simulink model "W06_P1"  (R2024b)
settings: Solver=ode4  StartTime=0  StopTime=T_final  FixedStep=h  RelTol=1e-3
undefined symbols (not defined in the file or in its folder): beta_c, mp, N_SEQ, rp, T_SW, V_c, x0, X_SEQ
settings Model: Creator=admin  LastModifiedBy=admin
settings DataIOCC: ReturnWorkspaceOutputs=off

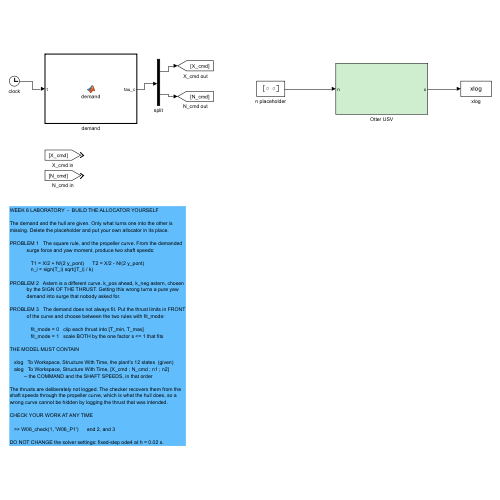
[thumbnail: Simulink's stored preview of the top-level diagram]
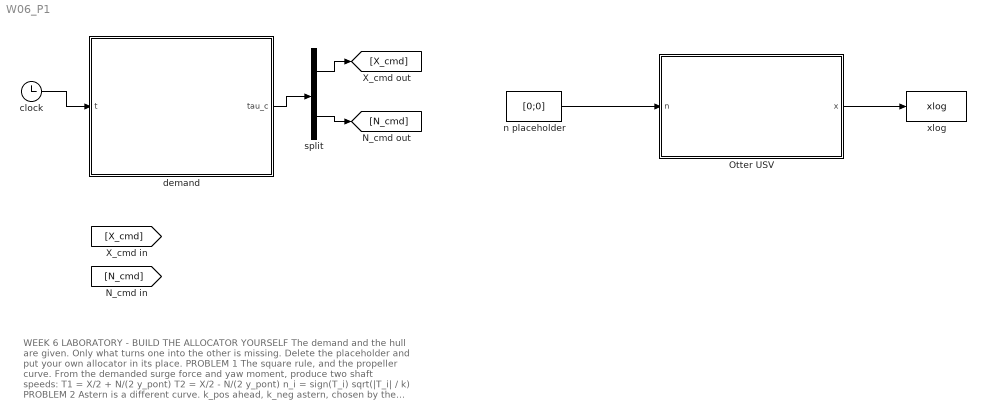
== system W06_P1 ==
  note: WEEK 6 LABORATORY  -  BUILD THE ALLOCATOR YOURSELF
      |
      | The demand and the hull are given. Only what turns one into the other is
      | missing. Delete the placeholder and put your own allocator in its place.
      |
      | PROBLEM 1   The square rule, and the propeller curve. From the demanded
      |             surge force and yaw moment, produce two shaft speeds:
      |
      |                T1 = X/2 + N/(2 y_pont)      T2 = X/2 - N/(2 y_pont)
      |                n_i = sign(T_i) sqrt(|T_i| / k)
      |
      | PROBLEM 2   Astern is a different curve. k_pos ahead, k_neg astern, chosen
      |             by the SIGN OF THE THRUST. Getting this wrong turns a pure yaw
      |             demand into surge that nobody asked for.
      |
      | PROBLEM 3   The demand does not always fit. Put the thrust limits in FRONT
      |             of the curve and choose between the two rules with fit_mode:
      |
      |                fit_mode = 0   clip each thrust into [T_min, T_max]
      |                fit_mode = 1   scale BOTH by the one factor s <= 1 that fits
      |
      | THE MODEL MUST CONTAIN
      |
      |    xlog   To Workspace, Structure With Time, the plant's 12 states  (given)
      |    alog   To Workspace, Structure With Time, [X_cmd ; N_cmd ; n1 ; n2]
      |           -- the COMMAND and the SHAFT SPEEDS, in that order
      |
      | The thrusts are deliberately not logged. The checker recovers them from the
      | shaft speeds through the propeller curve, which is what the hull does, so a
      | wrong curve cannot be hidden by logging the thrust that was intended.
      |
      | CHECK YOUR WORK AT ANY TIME
      |
      |    >> W06_check(1, 'W06_P1')      and 2, and 3
      |
      | DO NOT CHANGE the solver settings: fixed-step ode4 at h = 0.02 s.
  Otter USV : Subsystem
  clock : Clock
  demand : MATLAB Function  TreatAsAtomicUnit=on
  n placeholder : Constant  Value=[0;0]
  split : Demux  Outputs=2
  xlog : ToWorkspace  VariableName=xlog  SaveFormat=Structure With Time  SampleTime=-1
  wires:
  clock/1 -> demand/1(t)
  demand/1(tau_c) -> split/1
  split/1 -> [X_cmd]
  split/2 -> [N_cmd]
  Otter USV/1(x) -> xlog/1
  n placeholder/1 -> Otter USV/1(n)

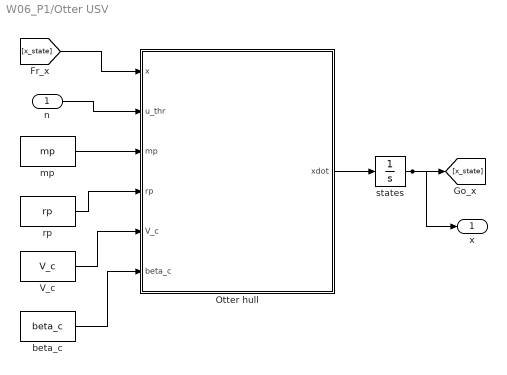
== system W06_P1/Otter USV ==
  n : Inport
  Otter hull : MATLAB Function  TreatAsAtomicUnit=on
  V_c : Constant  Value=V_c
  beta_c : Constant  Value=beta_c
  mp : Constant  Value=mp
  rp : Constant  Value=rp
  states : Integrator  InitialCondition=x0
  x : Outport
  wires:
  n/1 -> Otter hull/2(u_thr)
  [x_state] -> Otter hull/1(x)
  mp/1 -> Otter hull/3(mp)
  rp/1 -> Otter hull/4(rp)
  V_c/1 -> Otter hull/5(V_c)
  Otter hull/1(xdot) -> states/1
  beta_c/1 -> Otter hull/6(beta_c)
  states/1 -> [x_state], x/1

== matlab function W06_P1/Otter USV/Otter hull ==
  data: x input; xdot output double size=[12 1]; u_thr input; mp input; rp input; V_c input; beta_c input
function xdot = otter_hull(x, u_thr, mp, rp, V_c, beta_c)
% Fossen's otter.m, called unchanged from Tools/MSS/VESSELS.
%
%   x       12 states, fed back from the integrator
%   u_thr   propeller shaft speeds [rad/s]
%
% otter.m is not written for code generation, so the call is extrinsic and
% xdot has to be pre-sized for Simulink to know the output width.
coder.extrinsic('otter');

xdot = zeros(12,1);
xdot = otter(x, u_thr, mp, rp, V_c, beta_c);
end

== matlab function W06_P1/demand ==
  data: t input; tau_c output double size=[2 1]; T_SW parameter; X_SEQ parameter; N_SEQ parameter
function tau_c = demand(t, T_SW, X_SEQ, N_SEQ)
%#codegen
%DEMAND  요구 시간표 / the demand timetable.
%
%  T_SW(i) 초부터 (X_SEQ(i), N_SEQ(i)) 를 요구한다. 세 벡터는 워크스페이스에
%  있고, W06_check 가 문제마다 다시 넣는다.
%  From T_SW(i) seconds the demand is (X_SEQ(i), N_SEQ(i)). The three vectors
%  live in the workspace and W06_check sets them for each problem.
k = 1;
for i = 1:numel(T_SW)
    if t >= T_SW(i), k = i; end
end
tau_c = [X_SEQ(k); N_SEQ(k)];
